simulink model "ForwardDynamics_harmonic"  (Simulink 8.7)
settings: Solver=ode45  StartTime=0.0  StopTime=4  RelTol=1e-3
settings Model: Creator=gwu  LastModifiedBy=Guilherme
settings DataIOCC: SignalLoggingSaveFormat=ModelDataLogs
settings OptimizationCC: ExpressionDepthLimit=2147483647
settings DebuggingCC: SolverPrmCheckMsg=warning  FcnCallInpInsideContextMsg=EnableAllAsWarning  StateNameClashWarn=warning
settings RTWCC: TargetLang=C++

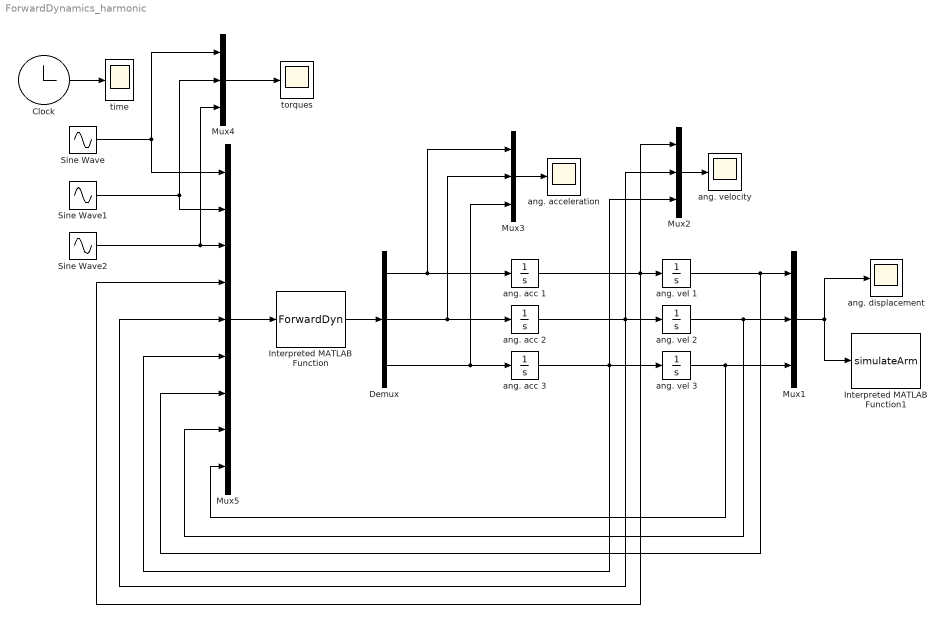
== system ForwardDynamics_harmonic ==
  Clock : Clock
  Demux : Demux  Outputs=3
  Interpreted MATLAB Function : MATLABFcn  MATLABFcn=ForwardDyn  OutputDimensions=3  OutputSignalType=real
  Interpreted MATLAB Function1 : MATLABFcn  MATLABFcn=simulateArm  OutputDimensions=0
  Mux{1..4} (4 alike) : Mux  Inputs=3
  Mux5 : Mux  Inputs=9
  Sine Wave : Sin  Amplitude=-5  Frequency=0.5*pi  SampleTime=0
  Sine Wave1 : Sin  Amplitude=-2  Frequency=pi  SampleTime=0
  Sine Wave2 : Sin  Amplitude=-2  Frequency=pi  SampleTime=0
  ang. acc 1 : Integrator
  ang. acc 2 : Integrator
  ang. acc 3 : Integrator
  ang. acceleration : Scope
  ang. displacement : Scope
  ang. vel 1 : Integrator
  ang. vel 2 : Integrator
  ang. vel 3 : Integrator
  ang. velocity : Scope
  time : Scope
  torques : Scope
  wires:
  ang. acc 1/1 -> Mux5/4, ang. vel 1/1, Mux2/1
  ang. vel 1/1 -> Mux5/7, Mux1/1
  ang. vel 2/1 -> Mux5/8, Mux1/2
  ang. acc 2/1 -> Mux5/5, ang. vel 2/1, Mux2/2
  Sine Wave/1 -> Mux5/1, Mux4/1
  Sine Wave1/1 -> Mux5/2, Mux4/2
  Interpreted MATLAB Function/1 -> Demux/1
  Demux/1 -> ang. acc 1/1, Mux3/1
  Demux/2 -> ang. acc 2/1, Mux3/2
  Mux1/1 -> ang. displacement/1, Interpreted MATLAB Function1/1
  Mux2/1 -> ang. velocity/1
  Mux3/1 -> ang. acceleration/1
  Clock/1 -> time/1
  Mux4/1 -> torques/1
  Mux5/1 -> Interpreted MATLAB Function/1
  Sine Wave2/1 -> Mux4/3, Mux5/3
  Demux/3 -> Mux3/3, ang. acc 3/1
  ang. acc 3/1 -> Mux5/6, Mux2/3, ang. vel 3/1
  ang. vel 3/1 -> Mux5/9, Mux1/3
